simulink model "MPCApollo"  (Simulink 9.3)
settings: Solver=FixedStepAuto  StartTime=0  StopTime=inf  FixedStep=0.01  RelTol=1e-3  AbsTol=1e-6
model workspace (MAT data in the model file):
  SL_ROS_VariableLengthArrays_MaxSizes.CommonInfo.ArrayTruncateAction = 'EmitWarning'
  SL_ROS_VariableLengthArrays_MaxSizes.MsgTypeMap = containers.Map
  SL_ROS_VariableLengthArrays_MaxSizes.MsgTypeMap.serialization.keys = {'pnc_msgs/Trajectory'}
  SL_ROS_VariableLengthArrays_MaxSizes.MsgTypeMap.serialization.values{1}.PropertyName = 'TrajectoryPts'
  SL_ROS_VariableLengthArrays_MaxSizes.MsgTypeMap.serialization.values{1}.DataType = 'pnc_msgs/TrajectoryPoint'
  SL_ROS_VariableLengthArrays_MaxSizes.MsgTypeMap.serialization.values{1}.MaxLength = 359
  SL_ROS_VariableLengthArrays_MaxSizes.MsgTypeMap.serialization.uniformity = 0
  SL_ROS_VariableLengthArrays_MaxSizes.MsgTypeMap.serialization.keyType = 'char'
  SL_ROS_VariableLengthArrays_MaxSizes.MsgTypeMap.serialization.valueType = 'any'
libraries: simulink x1, Solver_SF x1
settings Model: Creator=pmather  LastModifiedBy=ck_le  SimulationMode=accelerator  ExtModeTrigMode=oneshot  ExtModeArmWhenConnect=off
settings SolverCC: AutoScaleAbsTol=off
settings DataIOCC: SignalLoggingName=sigsOut
settings OptimizationCC: BlockReduction=off  BooleanDataType=off  ExpressionDepthLimit=2147483647
settings DebuggingCC: SaveWithParameterizedLinksMsg=none  SignalResolutionControl=TryResolveAllWithWarning  MultiTaskDSMMsg=warning  MultiTaskCondExecSysMsg=none  StateNameClashWarn=warning
settings HardwareCC: TargetUnknown=on
settings RTWCC: TemplateMakefile=grt_vc.tmf
settings GRTTargetCC: GeneratePreprocessorConditionals=Disable all

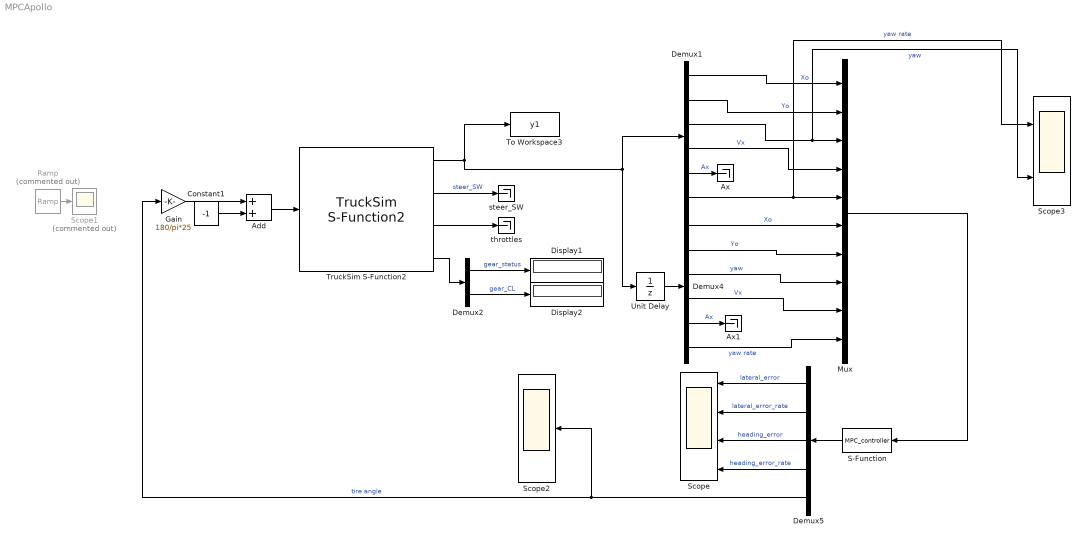
== system MPCApollo ==
  Add : Sum
  Ax : Terminator
  Ax1 : Terminator
  Constant1 : Constant  Value=-1
  Demux1 : Demux  Outputs=6
  Demux2 : Demux  Outputs=2
  Demux4 : Demux  Outputs=6
  Demux5 : Demux  Outputs=5
  Display1 : Display
  Display2 : Display
  Gain : Gain  Gain=180/pi*25
  Mux : Mux  Inputs=10
  Ramp : simulink/Sources/Ramp  Commented=on  slope=100  start=0  InitialOutput=0
  S-Function : S-Function  FunctionName=MPC_controller  SFunctionDeploymentMode=off  EnableBusSupport=off
  Scope : Scope  NumInputPorts=4
  Scope1 : Scope  Commented=on
  Scope2 : Scope
  Scope3 : Scope  NumInputPorts=2
  To Workspace3 : ToWorkspace  VariableName=y1  SaveFormat=Timeseries  SampleTime=-1
  TruckSim S-Function2 : Solver_SF/TruckSim S-Function2  Priority=1  VehicleCode=s_s  SIMFILE=simfile.sim
      settings: AttributesFormatString=Vehicle Code: %<VehicleCode>
  Unit Delay : UnitDelay  SampleTime=-1  HasFrameUpgradeWarning=on
  steer_SW : Terminator
  throttles : Terminator
  wires:
  TruckSim S-Function2/1 -> To Workspace3/1, Unit Delay/1, Demux1/1
  Demux1/4 -> Mux/4  "Vx"
  Demux1/6 -> Scope3/1, Mux/5  "yaw rate"
  Demux2/1 -> Display1/1  "gear_status"
  Demux2/2 -> Display2/1  "gear_CL"
  TruckSim S-Function2/2 -> steer_SW/1  "steer_SW"
  TruckSim S-Function2/3 -> throttles/1
  TruckSim S-Function2/4 -> Demux2/1
  Demux1/3 -> Scope3/2, Mux/3  "yaw"
  Unit Delay/1 -> Demux4/1
  Demux4/1 -> Mux/6  "Xo"
  Demux4/2 -> Mux/7  "Yo"
  Demux4/3 -> Mux/8  "yaw"
  Demux4/4 -> Mux/9  "Vx"
  Demux4/5 -> Ax1/1  "Ax"
  Demux4/6 -> Mux/10  "yaw rate"
  Demux1/5 -> Ax/1  "Ax"
  Demux1/2 -> Mux/2  "Yo"
  Demux1/1 -> Mux/1  "Xo"
  Mux/1 -> S-Function/1
  S-Function/1 -> Demux5/1
  Demux5/5 -> Scope2/1, Gain/1  "tire angle"
  Demux5/3 -> Scope/3  "heading_error"
  Demux5/2 -> Scope/2  "lateral_error_rate"
  Demux5/1 -> Scope/1  "lateral_error"
  Demux5/4 -> Scope/4  "heading_error_rate"
  Ramp/1 -> Scope1/1
  Add/1 -> TruckSim S-Function2/1
  Constant1/1 -> Add/2
  Gain/1 -> Add/1
